simulink library "ammclib_bam_s32k11x"  (Simulink 9.0)
settings: Solver=ode45  StartTime=0.0  StopTime=10.0  RelTol=1e-3
undefined symbols (not defined in the file): f16A1, f16A2, f16B0, f16B1, f16B2, f16C1, f16CC1, f16CC1sc, f16CC1sc_D, f16CC1sc_Q, f16CC1scD, f16CC1scQ, f16CC2, f16CC2sc, f16CC2sc_D, f16CC2sc_Q, f16CC2scD, f16CC2scQ, f16DerivGain, f16EGain, f16FiltCoef, f16HystOff, f16HystOn, f16IGain, f16IntegGain, f16IntegGainFW, f16IntegGainQ, f16Kd, f16Kq, f16Limit, f16LowerLim, f16LowerLimit_D, f16LowerLimit_Q, f16ModIndex, f16OutValOff, f16OutValOn, f16PropGain, f16PropGainFW, f16PropGainQ, f16RampDown, f16RampUp, f16UGain, f16UpperLim, f16UpperLimit, f16UpperLimit_D, f16UpperLimit_Q, f16WIGain, f32A1, f32A2, f32B0, f32B1, f32B2, f32C1, f32CC1, f32CC1sc, f32CC1sc_D, f32CC1sc_Q, f32CC1scD, f32CC1scQ, f32CC2 ... (+71)
(part 6 of 7)

== system ammclib_bam_s32k11x/MLIB/bam_f16/MLIB_AddSat_F16 ==
  note: ---------------------------------------------------------------------------------------------------------------------------------------------------------------------------------------------------
  f16In1 : Inport
  f16In2 : Inport  Port=2
  MLIB_AddSat_SF : S-Function  FunctionName=MLIB_AddSat_SF_F16  SFunctionDeploymentMode=off  EnableBusSupport=off
  copyright : Subsystem
      mask Display:
      | text(10,90,'FILE:');text(10,75,'DESRIPTION:')
      | text(10,60,'COPYRIGHT:')
      | text(10,45,'VERSION:')
      | text(10,30,'DATE:')
  copyright2 : Subsystem
      mask Display:
      | text(10,90,'MLIB_AddSat_BAM_F16.mdl');text(10,75,'Saturated sum of two input values.');text(10,60,'NXP')
      | text(10,45,'0.1');text(10,30,'20-Jan-2012');
  logo : Subsystem
      mask Display: image(imread('logo.jpg'))
  f16Out : Outport
  wires:
  MLIB_AddSat_SF/1 -> f16Out/1
  f16In2/1 -> MLIB_AddSat_SF/2
  f16In1/1 -> MLIB_AddSat_SF/1

== system ammclib_bam_s32k11x/MLIB/bam_f16/MLIB_Add_F16 ==
  note: ---------------------------------------------------------------------------------------------------------------------------------------------------------------------------------------------------
  f16In1 : Inport
  f16In2 : Inport  Port=2
  MLIB_Add_SF : S-Function  FunctionName=MLIB_Add_SF_F16  SFunctionDeploymentMode=off  EnableBusSupport=off
  copyright : Subsystem
      mask Display:
      | text(10,90,'FILE:');text(10,75,'DESRIPTION:')
      | text(10,60,'COPYRIGHT:')
      | text(10,45,'VERSION:')
      | text(10,30,'DATE:')
  copyright2 : Subsystem
      mask Display:
      | text(10,90,'MLIB_Add_BAM_F16.mdl');text(10,75,'Sum of two input values.');text(10,60,'NXP')
      | text(10,45,'0.1');text(10,30,'20-Jan-2012');
  logo : Subsystem
      mask Display: image(imread('logo.jpg'))
  f16Out : Outport
  wires:
  MLIB_Add_SF/1 -> f16Out/1
  f16In2/1 -> MLIB_Add_SF/2
  f16In1/1 -> MLIB_Add_SF/1

== system ammclib_bam_s32k11x/MLIB/bam_f16/MLIB_ConvertPU_F16F32 ==
  note: ---------------------------------------------------------------------------------------------------------------------------------------------------------------------------------------------------
  f32In : Inport
  MLIB_ConvertPU_SF : S-Function  FunctionName=MLIB_ConvertPU_SF_F16F32  SFunctionDeploymentMode=off  EnableBusSupport=off
  copyright : Subsystem
      mask Display: text(10,90,'FILE:');text(10,75,'DESRIPTION:')text(10,60,'COPYRIGHT:')text(10,45,'VERSION:')text(10,30,'DATE:')
  copyright2 : Subsystem
      mask Display: text(10,90,'MLIB_ConvertPU_BAM_F16.mdl');text(10,75,'Converts the input value to different representation in unity model.');text(10,60,'NXP')text(10,45,'0.1');text(10,30,'10-Oct-2011');
  logo : Subsystem
      mask Display: image(imread('logo.jpg'))
  f16Out : Outport
  wires:
  MLIB_ConvertPU_SF/1 -> f16Out/1
  f32In/1 -> MLIB_ConvertPU_SF/1

== system ammclib_bam_s32k11x/MLIB/bam_f16/MLIB_Convert_F16F32 ==
  note: ---------------------------------------------------------------------------------------------------------------------------------------------------------------------------------------------------
  f32In1 : Inport
  f32In2 : Inport  Port=2
  MLIB_Convert_SF : S-Function  FunctionName=MLIB_Convert_SF_F16F32  SFunctionDeploymentMode=off  EnableBusSupport=off
  copyright : Subsystem
      mask Display:
      | text(10,90,'FILE:');text(10,75,'DESRIPTION:')
      | text(10,60,'COPYRIGHT:')
      | text(10,45,'VERSION:')
      | text(10,30,'DATE:')
  copyright2 : Subsystem
      mask Display:
      | text(10,90,'MLIB_Convert_BAM_F16F32.mdl');text(10,75,'Converts the input value with scale to different representation in unity model.');text(10,60,'NXP')
      | text(10,45,'0.1');text(10,30,'13-Oct-2011');
  logo : Subsystem
      mask Display: image(imread('logo.jpg'))
  f16Out : Outport
  wires:
  MLIB_Convert_SF/1 -> f16Out/1
  f32In2/1 -> MLIB_Convert_SF/2
  f32In1/1 -> MLIB_Convert_SF/1

== system ammclib_bam_s32k11x/MLIB/bam_f16/MLIB_DivSat_F16 ==
  note: ---------------------------------------------------------------------------------------------------------------------------------------------------------------------------------------------------
  f16In1 : Inport
  f16In2 : Inport  Port=2
  MLIB_DivSat_SF : S-Function  FunctionName=MLIB_DivSat_SF_F16  SFunctionDeploymentMode=off  EnableBusSupport=off
  copyright : Subsystem
      mask Display:
      | text(10,90,'FILE:');text(10,75,'DESRIPTION:')
      | text(10,60,'COPYRIGHT:')
      | text(10,45,'VERSION:')
      | text(10,30,'DATE:')
  copyright2 : Subsystem
      mask Display:
      | text(10,90,'MLIB_DivSat_BAM_F16.mdl');text(10,75,'Division of two input values saturated if necessary.');text(10,60,'NXP')
      | text(10,45,'0.1');text(10,30,'19-Aug-2011');
  logo : Subsystem
      mask Display: image(imread('logo.jpg'))
  f16Out : Outport
  wires:
  MLIB_DivSat_SF/1 -> f16Out/1
  f16In2/1 -> MLIB_DivSat_SF/2
  f16In1/1 -> MLIB_DivSat_SF/1

== system ammclib_bam_s32k11x/MLIB/bam_f16/MLIB_Div_F16 ==
  note: ---------------------------------------------------------------------------------------------------------------------------------------------------------------------------------------------------
  f16In1 : Inport
  f16In2 : Inport  Port=2
  MLIB_Div_SF : S-Function  FunctionName=MLIB_Div_SF_F16  SFunctionDeploymentMode=off  EnableBusSupport=off
  copyright : Subsystem
      mask Display:
      | text(10,90,'FILE:');text(10,75,'DESRIPTION:')
      | text(10,60,'COPYRIGHT:')
      | text(10,45,'VERSION:')
      | text(10,30,'DATE:')
  copyright2 : Subsystem
      mask Display:
      | text(10,90,'MLIB_Div_BAM_F16.mdl');text(10,75,'Division of two input values.');text(10,60,'Freescale')
      | text(10,45,'0.1');text(10,30,'19-Aug-2011');
  logo : Subsystem
      mask Display: image(imread('logo.jpg'))
  f16Out : Outport
  wires:
  MLIB_Div_SF/1 -> f16Out/1
  f16In2/1 -> MLIB_Div_SF/2
  f16In1/1 -> MLIB_Div_SF/1

== system ammclib_bam_s32k11x/MLIB/bam_f16/MLIB_MacSat_F16 ==
  note: ---------------------------------------------------------------------------------------------------------------------------------------------------------------------------------------------------
  f16In1 : Inport
  f16In2 : Inport  Port=2
  f16In3 : Inport  Port=3
  MLIB_MacSat_SF : S-Function  FunctionName=MLIB_MacSat_SF_F16  SFunctionDeploymentMode=off  EnableBusSupport=off
  copyright : Subsystem
      mask Display:
      | text(10,90,'FILE:');text(10,75,'DESRIPTION:')
      | text(10,60,'COPYRIGHT:')
      | text(10,45,'VERSION:')
      | text(10,30,'DATE:')
  copyright2 : Subsystem
      mask Display:
      | text(10,90,'MLIB_MacSat_BAM_F16.mdl');text(10,75,'Saturated sum of two input values.');text(10,60,'NXP')
      | text(10,45,'0.1');text(10,30,'22-Aug-2011');
  logo : Subsystem
      mask Display: image(imread('logo.jpg'))
  f16Out : Outport
  wires:
  MLIB_MacSat_SF/1 -> f16Out/1
  f16In3/1 -> MLIB_MacSat_SF/3
  f16In2/1 -> MLIB_MacSat_SF/2
  f16In1/1 -> MLIB_MacSat_SF/1

== system ammclib_bam_s32k11x/MLIB/bam_f16/MLIB_Mac_F16 ==
  note: ---------------------------------------------------------------------------------------------------------------------------------------------------------------------------------------------------
  f16In1 : Inport
  f16In2 : Inport  Port=2
  f16In3 : Inport  Port=3
  MLIB_Mac_SF : S-Function  FunctionName=MLIB_Mac_SF_F16  SFunctionDeploymentMode=off  EnableBusSupport=off
  copyright : Subsystem
      mask Display:
      | text(10,90,'FILE:');text(10,75,'DESRIPTION:')
      | text(10,60,'COPYRIGHT:')
      | text(10,45,'VERSION:')
      | text(10,30,'DATE:')
  copyright2 : Subsystem
      mask Display:
      | text(10,90,'MLIB_Mac_BAM_F16.mdl');text(10,75,'Sum of two input values.');text(10,60,'NXP')
      | text(10,45,'0.1');text(10,30,'18-Jul-2011');
  logo : Subsystem
      mask Display: image(imread('logo.jpg'))
  f16Out : Outport
  wires:
  MLIB_Mac_SF/1 -> f16Out/1
  f16In3/1 -> MLIB_Mac_SF/3
  f16In2/1 -> MLIB_Mac_SF/2
  f16In1/1 -> MLIB_Mac_SF/1

== system ammclib_bam_s32k11x/MLIB/bam_f16/MLIB_Mnac_F16 ==
  note: ---------------------------------------------------------------------------------------------------------------------------------------------------------------------------------------------------
  f16In1 : Inport
  f16In2 : Inport  Port=2
  f16In3 : Inport  Port=3
  MLIB_Mnac_SF : S-Function  FunctionName=MLIB_Mnac_SF_F16  SFunctionDeploymentMode=off  EnableBusSupport=off
  copyright : Subsystem
      mask Display:
      | text(10,90,'FILE:');text(10,75,'DESRIPTION:')
      | text(10,60,'COPYRIGHT:')
      | text(10,45,'VERSION:')
      | text(10,30,'DATE:')
  copyright2 : Subsystem
      mask Display:
      | text(10,90,'MLIB_Mnac_BAM_F16.mdl');text(10,75,'Multiply-negative-accumulate.');text(10,60,'Freescale')
      | text(10,45,'1.0');text(10,30,'27-Mar-2015');
  logo : Subsystem
      mask Display: image(imread('logo.jpg'))
  f16Out : Outport
  wires:
  MLIB_Mnac_SF/1 -> f16Out/1
  f16In3/1 -> MLIB_Mnac_SF/3
  f16In2/1 -> MLIB_Mnac_SF/2
  f16In1/1 -> MLIB_Mnac_SF/1

== system ammclib_bam_s32k11x/MLIB/bam_f16/MLIB_Msu_F16 ==
  note: ---------------------------------------------------------------------------------------------------------------------------------------------------------------------------------------------------
  f16In1 : Inport
  f16In2 : Inport  Port=2
  f16In3 : Inport  Port=3
  MLIB_Msu_SF : S-Function  FunctionName=MLIB_Msu_SF_F16  SFunctionDeploymentMode=off  EnableBusSupport=off
  copyright : Subsystem
      mask Display:
      | text(10,90,'FILE:');text(10,75,'DESRIPTION:')
      | text(10,60,'COPYRIGHT:')
      | text(10,45,'VERSION:')
      | text(10,30,'DATE:')
  copyright2 : Subsystem
      mask Display:
      | text(10,90,'MLIB_Msu_BAM_F16.mdl');text(10,75,'Multiply-subtract-from.');text(10,60,'NXP')
      | text(10,45,'1.0');text(10,30,'27-Mar-2015');
  logo : Subsystem
      mask Display: image(imread('logo.jpg'))
  f16Out : Outport
  wires:
  MLIB_Msu_SF/1 -> f16Out/1
  f16In3/1 -> MLIB_Msu_SF/3
  f16In2/1 -> MLIB_Msu_SF/2
  f16In1/1 -> MLIB_Msu_SF/1

== system ammclib_bam_s32k11x/MLIB/bam_f16/MLIB_MulSat_F16 ==
  note: ---------------------------------------------------------------------------------------------------------------------------------------------------------------------------------------------------
  f16In1 : Inport
  f16In2 : Inport  Port=2
  MLIB_MulSat_SF : S-Function  FunctionName=MLIB_MulSat_SF_F16  SFunctionDeploymentMode=off  EnableBusSupport=off
  copyright : Subsystem
      mask Display:
      | text(10,90,'FILE:');text(10,75,'DESRIPTION:')
      | text(10,60,'COPYRIGHT:')
      | text(10,45,'VERSION:')
      | text(10,30,'DATE:')
  copyright2 : Subsystem
      mask Display:
      | text(10,90,'MLIB_MulSat_BAM_F16.mdl');text(10,75,'Saturated sum of two input values.');text(10,60,'NXP')
      | text(10,45,'0.1');text(10,30,'01-Aug-2011');
  logo : Subsystem
      mask Display: image(imread('logo.jpg'))
  f16Out : Outport
  wires:
  MLIB_MulSat_SF/1 -> f16Out/1
  f16In2/1 -> MLIB_MulSat_SF/2
  f16In1/1 -> MLIB_MulSat_SF/1

== system ammclib_bam_s32k11x/MLIB/bam_f16/MLIB_Mul_F16 ==
  note: ---------------------------------------------------------------------------------------------------------------------------------------------------------------------------------------------------
  f16In1 : Inport
  f16In2 : Inport  Port=2
  MLIB_Mul_SF : S-Function  FunctionName=MLIB_Mul_SF_F16  SFunctionDeploymentMode=off  EnableBusSupport=off
  copyright : Subsystem
      mask Display:
      | text(10,90,'FILE:');text(10,75,'DESRIPTION:')
      | text(10,60,'COPYRIGHT:')
      | text(10,45,'VERSION:')
      | text(10,30,'DATE:')
  copyright2 : Subsystem
      mask Display:
      | text(10,90,'MLIB_Mul_BAM_F16.mdl');text(10,75,'Sum of two input values.');text(10,60,'NXP')
      | text(10,45,'0.1');text(10,30,'26-Jul-2011');
  logo : Subsystem
      mask Display: image(imread('logo.jpg'))
  f16Out : Outport
  wires:
  MLIB_Mul_SF/1 -> f16Out/1
  f16In2/1 -> MLIB_Mul_SF/2
  f16In1/1 -> MLIB_Mul_SF/1

== system ammclib_bam_s32k11x/MLIB/bam_f16/MLIB_NegSat_F16 ==
  note: ---------------------------------------------------------------------------------------------------------------------------------------------------------------------------------------------------
  f16In : Inport
  MLIB_NegSat_SF : S-Function  FunctionName=MLIB_NegSat_SF_F16  SFunctionDeploymentMode=off  EnableBusSupport=off
  copyright : Subsystem
      mask Display: text(10,90,'FILE:');text(10,75,'DESRIPTION:')text(10,60,'COPYRIGHT:')text(10,45,'VERSION:')text(10,30,'DATE:')
  copyright2 : Subsystem
      mask Display: text(10,90,'MLIB_NegSat_BAM_F16.mdl');text(10,75,'Sum of two input values.');text(10,60,'NXP')text(10,45,'0.1');text(10,30,'12-Jul-2011');
  logo : Subsystem
      mask Display: image(imread('logo.jpg'))
  f16Out : Outport
  wires:
  MLIB_NegSat_SF/1 -> f16Out/1
  f16In/1 -> MLIB_NegSat_SF/1

== system ammclib_bam_s32k11x/MLIB/bam_f16/MLIB_Neg_F16 ==
  note: ---------------------------------------------------------------------------------------------------------------------------------------------------------------------------------------------------
  f16In : Inport
  MLIB_Neg_SF : S-Function  FunctionName=MLIB_Neg_SF_F16  SFunctionDeploymentMode=off  EnableBusSupport=off
  copyright : Subsystem
      mask Display: text(10,90,'FILE:');text(10,75,'DESRIPTION:')text(10,60,'COPYRIGHT:')text(10,45,'VERSION:')text(10,30,'DATE:')
  copyright2 : Subsystem
      mask Display: text(10,90,'MLIB_Neg_BAM_F16.mdl');text(10,75,'Sum of two input values.');text(10,60,'NXP')text(10,45,'0.1');text(10,30,'20-Jan-2012');
  logo : Subsystem
      mask Display: image(imread('logo.jpg'))
  f16Out : Outport
  wires:
  MLIB_Neg_SF/1 -> f16Out/1
  f16In/1 -> MLIB_Neg_SF/1

== system ammclib_bam_s32k11x/MLIB/bam_f16/MLIB_Norm_F16 ==
  note: ---------------------------------------------------------------------------------------------------------------------------------------------------------------------------------------------------
  f16In : Inport
  MLIB_Norm_SF_F16 : S-Function  FunctionName=MLIB_Norm_SF_F16  SFunctionDeploymentMode=off  EnableBusSupport=off
  copyright : Subsystem
      mask Display: text(10,90,'FILE:');text(10,75,'DESRIPTION:')text(10,60,'COPYRIGHT:')text(10,45,'VERSION:')text(10,30,'DATE:')
  copyright2 : Subsystem
      mask Display: text(10,90,'MLIB_Norm_BAM_F16.mdl');text(10,75,'Normalization of the input value.');text(10,60,'Freescale')text(10,45,'0.1');text(10,30,'15-Sep-2011');
  logo : Subsystem
      mask Display: image(imread('logo.jpg'))
  u16Out : Outport
  wires:
  MLIB_Norm_SF_F16/1 -> u16Out/1
  f16In/1 -> MLIB_Norm_SF_F16/1

== system ammclib_bam_s32k11x/MLIB/bam_f16/MLIB_RndSat_F16F32 ==
  note: ---------------------------------------------------------------------------------------------------------------------------------------------------------------------------------------------------
  f32In : Inport
  MLIB_RndSat_SF : S-Function  FunctionName=MLIB_RndSat_SF_F16F32  SFunctionDeploymentMode=off  EnableBusSupport=off
  copyright : Subsystem
      mask Display: text(10,90,'FILE:');text(10,75,'DESRIPTION:');text(10,60,'COPYRIGHT:');text(10,45,'VERSION:');text(10,30,'DATE:')
  copyright2 : Subsystem
      mask Display: text(10,90,'MLIB_RndSat_BAM_F16F32.mdl');text(10,75,'Rounding of the input value to the nearest saturated value in output format.');text(10,60,'NXP');text(10,45,'1.0');text(10,30,'05-May-2016');
  logo : Subsystem
      mask Display: image(imread('logo.jpg'))
  f16Out : Outport
  wires:
  MLIB_RndSat_SF/1 -> f16Out/1
  f32In/1 -> MLIB_RndSat_SF/1

== system ammclib_bam_s32k11x/MLIB/bam_f16/MLIB_Round_F16 ==
  note: ---------------------------------------------------------------------------------------------------------------------------------------------------------------------------------------------------
  f16In1 : Inport
  u16In2 : Inport  Port=2
  MLIB_Round_SF_F16 : S-Function  FunctionName=MLIB_Round_SF_F16  SFunctionDeploymentMode=off  EnableBusSupport=off
  copyright : Subsystem
      mask Display:
      | text(10,90,'FILE:');text(10,75,'DESRIPTION:')
      | text(10,60,'COPYRIGHT:')
      | text(10,45,'VERSION:')
      | text(10,30,'DATE:')
  copyright2 : Subsystem
      mask Display:
      | text(10,90,'MLIB_Round_BAM_F16.mdl');text(10,75,'Round the first input value.');text(10,60,'Freescale')
      | text(10,45,'0.1');text(10,30,'02-Sep-2011');
  logo : Subsystem
      mask Display: image(imread('logo.jpg'))
  f16Out : Outport
  wires:
  MLIB_Round_SF_F16/1 -> f16Out/1
  u16In2/1 -> MLIB_Round_SF_F16/2
  f16In1/1 -> MLIB_Round_SF_F16/1

== system ammclib_bam_s32k11x/MLIB/bam_f16/MLIB_ShBiSat_F16 ==
  note: ---------------------------------------------------------------------------------------------------------------------------------------------------------------------------------------------------
  f16In1 : Inport
  s16In2 : Inport  Port=2
  MLIB_ShBiSat_SF_F16 : S-Function  FunctionName=MLIB_ShBiSat_SF_F16  SFunctionDeploymentMode=off  EnableBusSupport=off
  copyright : Subsystem
      mask Display:
      | text(10,90,'FILE:');text(10,75,'DESRIPTION:')
      | text(10,60,'COPYRIGHT:')
      | text(10,45,'VERSION:')
      | text(10,30,'DATE:')
  copyright2 : Subsystem
      mask Display:
      | text(10,90,'MLIB_ShBiSat_BAM_F16.mdl');text(10,75,'Shift the first parameter to left or right and saturate if necessary.');text(10,60,'NXP')
      | text(10,45,'0.1');text(10,30,'26-Aug-2011');
  logo : Subsystem
      mask Display: image(imread('logo.jpg'))
  f16Out : Outport
  wires:
  MLIB_ShBiSat_SF_F16/1 -> f16Out/1
  s16In2/1 -> MLIB_ShBiSat_SF_F16/2
  f16In1/1 -> MLIB_ShBiSat_SF_F16/1

== system ammclib_bam_s32k11x/MLIB/bam_f16/MLIB_ShBi_F16 ==
  note: ---------------------------------------------------------------------------------------------------------------------------------------------------------------------------------------------------
  f16In1 : Inport
  s16In2 : Inport  Port=2
  MLIB_ShBi_SF_F16 : S-Function  FunctionName=MLIB_ShBi_SF_F16  SFunctionDeploymentMode=off  EnableBusSupport=off
  copyright : Subsystem
      mask Display:
      | text(10,90,'FILE:');text(10,75,'DESRIPTION:')
      | text(10,60,'COPYRIGHT:')
      | text(10,45,'VERSION:')
      | text(10,30,'DATE:')
  copyright2 : Subsystem
      mask Display:
      | text(10,90,'MLIB_ShBi_BAM_F16.mdl');text(10,75,'Shift the first parameter to left or right.');text(10,60,'NXP')
      | text(10,45,'0.1');text(10,30,'24-Aug-2011');
  logo : Subsystem
      mask Display: image(imread('logo.jpg'))
  f16Out : Outport
  wires:
  MLIB_ShBi_SF_F16/1 -> f16Out/1
  s16In2/1 -> MLIB_ShBi_SF_F16/2
  f16In1/1 -> MLIB_ShBi_SF_F16/1

== system ammclib_bam_s32k11x/MLIB/bam_f16/MLIB_ShLSat_F16 ==
  note: ---------------------------------------------------------------------------------------------------------------------------------------------------------------------------------------------------
  f16In1 : Inport
  u16In2 : Inport  Port=2
  MLIB_ShLSat_SF : S-Function  FunctionName=MLIB_ShLSat_SF_F16  SFunctionDeploymentMode=off  EnableBusSupport=off
  copyright : Subsystem
      mask Display:
      | text(10,90,'FILE:');text(10,75,'DESRIPTION:')
      | text(10,60,'COPYRIGHT:')
      | text(10,45,'VERSION:')
      | text(10,30,'DATE:')
  copyright2 : Subsystem
      mask Display:
      | text(10,90,'MLIB_ShLSat_BAM_F16.mdl');text(10,75,'Shift the first parameter to left and saturate if necessary.');text(10,60,'NXP')
      | text(10,45,'0.1');text(10,30,'19-Jul-2011');
  logo : Subsystem
      mask Display: image(imread('logo.jpg'))
  f16Out : Outport
  wires:
  MLIB_ShLSat_SF/1 -> f16Out/1
  u16In2/1 -> MLIB_ShLSat_SF/2
  f16In1/1 -> MLIB_ShLSat_SF/1

== system ammclib_bam_s32k11x/MLIB/bam_f16/MLIB_ShL_F16 ==
  note: ---------------------------------------------------------------------------------------------------------------------------------------------------------------------------------------------------
  f16In1 : Inport
  u16In2 : Inport  Port=2
  MLIB_ShL_SF_F16 : S-Function  FunctionName=MLIB_ShL_SF_F16  SFunctionDeploymentMode=off  EnableBusSupport=off
  copyright : Subsystem
      mask Display:
      | text(10,90,'FILE:');text(10,75,'DESRIPTION:')
      | text(10,60,'COPYRIGHT:')
      | text(10,45,'VERSION:')
      | text(10,30,'DATE:')
      | text(10,15,'AUTHOR:')
  copyright2 : Subsystem
      mask Display:
      | text(10,90,'MLIB_ShL_BAM_F16.mdl');text(10,75,'Shift the first parameter to left.');text(10,60,'Freescale')
      | text(10,45,'0.1');text(10,30,'04-Jul-2011');text(10,15,'');
  logo : Subsystem
      mask Display: image(imread('logo.jpg'))
  f16Out : Outport
  wires:
  u16In2/1 -> MLIB_ShL_SF_F16/2
  MLIB_ShL_SF_F16/1 -> f16Out/1
  f16In1/1 -> MLIB_ShL_SF_F16/1

== system ammclib_bam_s32k11x/MLIB/bam_f16/MLIB_ShR_F16 ==
  note: ---------------------------------------------------------------------------------------------------------------------------------------------------------------------------------------------------
  f16In1 : Inport
  u16In2 : Inport  Port=2
  MLIB_ShR_SF : S-Function  FunctionName=MLIB_ShR_SF_F16  SFunctionDeploymentMode=off  EnableBusSupport=off
  copyright : Subsystem
      mask Display:
      | text(10,90,'FILE:');text(10,75,'DESRIPTION:')
      | text(10,60,'COPYRIGHT:')
      | text(10,45,'VERSION:')
      | text(10,30,'DATE:')
  copyright2 : Subsystem
      mask Display:
      | text(10,90,'MLIB_ShR_BAM_F16.mdl');text(10,75,'Shift the first parameter to right.');text(10,60,'Freescale')
      | text(10,45,'0.1');text(10,30,'20-Jul-2011');
  logo : Subsystem
      mask Display: image(imread('logo.jpg'))
  f16Out : Outport
  wires:
  MLIB_ShR_SF/1 -> f16Out/1
  u16In2/1 -> MLIB_ShR_SF/2
  f16In1/1 -> MLIB_ShR_SF/1

== system ammclib_bam_s32k11x/MLIB/bam_f16/MLIB_SubSat_F16 ==
  note: ---------------------------------------------------------------------------------------------------------------------------------------------------------------------------------------------------
  f16In1 : Inport
  f16In2 : Inport  Port=2
  MLIB_SubSat_SF : S-Function  FunctionName=MLIB_SubSat_SF_F16  SFunctionDeploymentMode=off  EnableBusSupport=off
  copyright : Subsystem
      mask Display:
      | text(10,90,'FILE:');text(10,75,'DESRIPTION:')
      | text(10,60,'COPYRIGHT:')
      | text(10,45,'VERSION:')
      | text(10,30,'DATE:')
  copyright2 : Subsystem
      mask Display:
      | text(10,90,'MLIB_SubSat_BAM_F16.mdl');text(10,75,'Saturated sum of two input values.');text(10,60,'NXP')
      | text(10,45,'0.1');text(10,30,'20-Jan-2012');
  logo : Subsystem
      mask Display: image(imread('logo.jpg'))
  f16Out : Outport
  wires:
  MLIB_SubSat_SF/1 -> f16Out/1
  f16In2/1 -> MLIB_SubSat_SF/2
  f16In1/1 -> MLIB_SubSat_SF/1

== system ammclib_bam_s32k11x/MLIB/bam_f16/MLIB_Sub_F16 ==
  note: ---------------------------------------------------------------------------------------------------------------------------------------------------------------------------------------------------
  f16In1 : Inport
  f16In2 : Inport  Port=2
  MLIB_Sub_SF : S-Function  FunctionName=MLIB_Sub_SF_F16  SFunctionDeploymentMode=off  EnableBusSupport=off
  copyright : Subsystem
      mask Display:
      | text(10,90,'FILE:');text(10,75,'DESRIPTION:')
      | text(10,60,'COPYRIGHT:')
      | text(10,45,'VERSION:')
      | text(10,30,'DATE:')
  copyright2 : Subsystem
      mask Display:
      | text(10,90,'MLIB_Sub_BAM_F16.mdl');text(10,75,'Sum of two input values.');text(10,60,'NXP')
      | text(10,45,'0.1');text(10,30,'18-Jul-2011');
  logo : Subsystem
      mask Display: image(imread('logo.jpg'))
  f16Out : Outport
  wires:
  MLIB_Sub_SF/1 -> f16Out/1
  f16In2/1 -> MLIB_Sub_SF/2
  f16In1/1 -> MLIB_Sub_SF/1

== system ammclib_bam_s32k11x/MLIB/bam_f16/MLIB_VMac_F16 ==
  note: ---------------------------------------------------------------------------------------------------------------------------------------------------------------------------------------------------
  f16In1 : Inport
  f16In2 : Inport  Port=2
  f16In3 : Inport  Port=3
  f16In4 : Inport  Port=4
  MLIB_VMac_SF : S-Function  FunctionName=MLIB_VMac_SF_F16  SFunctionDeploymentMode=off  EnableBusSupport=off
  copyright : Subsystem
      mask Display:
      | text(10,90,'FILE:');text(10,75,'DESRIPTION:')
      | text(10,60,'COPYRIGHT:')
      | text(10,45,'VERSION:')
      | text(10,30,'DATE:')
  copyright2 : Subsystem
      mask Display:
      | text(10,90,'MLIB_VMac_BAM_F16.mdl');text(10,75,'Vector multiply accumulate.');text(10,60,'Freescale')
      | text(10,45,'0.1');text(10,30,'25-Aug-2011');
  logo : Subsystem
      mask Display: image(imread('logo.jpg'))
  f16Out : Outport
  wires:
  MLIB_VMac_SF/1 -> f16Out/1
  f16In4/1 -> MLIB_VMac_SF/4
  f16In3/1 -> MLIB_VMac_SF/3
  f16In2/1 -> MLIB_VMac_SF/2
  f16In1/1 -> MLIB_VMac_SF/1

== system ammclib_bam_s32k11x/MLIB/bam_f32/MLIB_AbsSat_F32 ==
  note: ---------------------------------------------------------------------------------------------------------------------------------------------------------------------------------------------------
  f32In : Inport
  MLIB_AbsSat_SF : S-Function  FunctionName=MLIB_AbsSat_SF_F32  SFunctionDeploymentMode=off  EnableBusSupport=off
  copyright : Subsystem
      mask Display: text(10,90,'FILE:');text(10,75,'DESRIPTION:')text(10,60,'COPYRIGHT:')text(10,45,'VERSION:')text(10,30,'DATE:')
  copyright2 : Subsystem
      mask Display: text(10,90,'MLIB_AbsSat_BAM_F32.mdl');text(10,75,'Absolute value of input parameter saturated if necessary.');text(10,60,'NXP')text(10,45,'0.1');text(10,30,'19-Aug-2011');
  logo : Subsystem
      mask Display: image(imread('logo.jpg'))
  f32Out : Outport
  wires:
  MLIB_AbsSat_SF/1 -> f32Out/1
  f32In/1 -> MLIB_AbsSat_SF/1

== system ammclib_bam_s32k11x/MLIB/bam_f32/MLIB_Abs_F32 ==
  note: ---------------------------------------------------------------------------------------------------------------------------------------------------------------------------------------------------
  f32In : Inport
  MLIB_Abs_SF : S-Function  FunctionName=MLIB_Abs_SF_F32  SFunctionDeploymentMode=off  EnableBusSupport=off
  copyright : Subsystem
      mask Display: text(10,90,'FILE:');text(10,75,'DESRIPTION:')text(10,60,'COPYRIGHT:')text(10,45,'VERSION:')text(10,30,'DATE:')
  copyright2 : Subsystem
      mask Display: text(10,90,'MLIB_Abs_BAM_F32.mdl');text(10,75,'Absolute value of input parameter.');text(10,60,'Freescale')text(10,45,'0.1');text(10,30,'20-Jan-2012');
  logo : Subsystem
      mask Display: image(imread('logo.jpg'))
  f32Out : Outport
  wires:
  MLIB_Abs_SF/1 -> f32Out/1
  f32In/1 -> MLIB_Abs_SF/1

== system ammclib_bam_s32k11x/MLIB/bam_f32/MLIB_AddSat_F32 ==
  note: ---------------------------------------------------------------------------------------------------------------------------------------------------------------------------------------------------
  f32In1 : Inport
  f32In2 : Inport  Port=2
  MLIB_AddSat_SF : S-Function  FunctionName=MLIB_AddSat_SF_F32  SFunctionDeploymentMode=off  EnableBusSupport=off
  copyright : Subsystem
      mask Display:
      | text(10,90,'FILE:');text(10,75,'DESRIPTION:')
      | text(10,60,'COPYRIGHT:')
      | text(10,45,'VERSION:')
      | text(10,30,'DATE:')
  copyright2 : Subsystem
      mask Display:
      | text(10,90,'MLIB_AddSat_BAM_F32.mdl');text(10,75,'Saturated sum of two input values.');text(10,60,'NXP')
      | text(10,45,'0.1');text(10,30,'20-Jan-2012');
  logo : Subsystem
      mask Display: image(imread('logo.jpg'))
  f32Out : Outport
  wires:
  MLIB_AddSat_SF/1 -> f32Out/1
  f32In2/1 -> MLIB_AddSat_SF/2
  f32In1/1 -> MLIB_AddSat_SF/1

== system ammclib_bam_s32k11x/MLIB/bam_f32/MLIB_Add_F32 ==
  note: ---------------------------------------------------------------------------------------------------------------------------------------------------------------------------------------------------
  f32In1 : Inport
  f32In2 : Inport  Port=2
  MLIB_Add_SF : S-Function  FunctionName=MLIB_Add_SF_F32  SFunctionDeploymentMode=off  EnableBusSupport=off
  copyright : Subsystem
      mask Display:
      | text(10,90,'FILE:');text(10,75,'DESRIPTION:')
      | text(10,60,'COPYRIGHT:')
      | text(10,45,'VERSION:')
      | text(10,30,'DATE:')
  copyright2 : Subsystem
      mask Display:
      | text(10,90,'MLIB_Add_BAM_F32.mdl');text(10,75,'Sum of two input values.');text(10,60,'NXP')
      | text(10,45,'0.1');text(10,30,'20-Jan-2012');
  logo : Subsystem
      mask Display: image(imread('logo.jpg'))
  f32Out : Outport
  wires:
  MLIB_Add_SF/1 -> f32Out/1
  f32In2/1 -> MLIB_Add_SF/2
  f32In1/1 -> MLIB_Add_SF/1

== system ammclib_bam_s32k11x/MLIB/bam_f32/MLIB_ConvertPU_F32F16 ==
  note: ---------------------------------------------------------------------------------------------------------------------------------------------------------------------------------------------------
  f16In : Inport
  MLIB_ConvertPU_SF : S-Function  FunctionName=MLIB_ConvertPU_SF_F32F16  SFunctionDeploymentMode=off  EnableBusSupport=off
  copyright : Subsystem
      mask Display: text(10,90,'FILE:');text(10,75,'DESRIPTION:')text(10,60,'COPYRIGHT:')text(10,45,'VERSION:')text(10,30,'DATE:')
  copyright2 : Subsystem
      mask Display: text(10,90,'MLIB_ConvertPU_BAM_F32.mdl');text(10,75,'Converts the input value to different representation in unity model.');text(10,60,'NXP')text(10,45,'0.1');text(10,30,'10-Oct-2011');
  logo : Subsystem
      mask Display: image(imread('logo.jpg'))
  f32Out : Outport
  wires:
  MLIB_ConvertPU_SF/1 -> f32Out/1
  f16In/1 -> MLIB_ConvertPU_SF/1

== system ammclib_bam_s32k11x/MLIB/bam_f32/MLIB_Convert_F32F16 ==
  note: ---------------------------------------------------------------------------------------------------------------------------------------------------------------------------------------------------
  f16In1 : Inport
  f16In2 : Inport  Port=2
  MLIB_Convert_SF : S-Function  FunctionName=MLIB_Convert_SF_F32F16  SFunctionDeploymentMode=off  EnableBusSupport=off
  copyright : Subsystem
      mask Display:
      | text(10,90,'FILE:');text(10,75,'DESRIPTION:')
      | text(10,60,'COPYRIGHT:')
      | text(10,45,'VERSION:')
      | text(10,30,'DATE:')
  copyright2 : Subsystem
      mask Display:
      | text(10,90,'MLIB_Convert_BAM_F32F16.mdl');text(10,75,'Converts the input value with scale to different representation in unity model.');text(10,60,'NXP')
      | text(10,45,'0.1');text(10,30,'13-Oct-2011');
  logo : Subsystem
      mask Display: image(imread('logo.jpg'))
  f32Out : Outport
  wires:
  MLIB_Convert_SF/1 -> f32Out/1
  f16In2/1 -> MLIB_Convert_SF/2
  f16In1/1 -> MLIB_Convert_SF/1

== system ammclib_bam_s32k11x/MLIB/bam_f32/MLIB_DivSat_F32 ==
  note: ---------------------------------------------------------------------------------------------------------------------------------------------------------------------------------------------------
  f32In1 : Inport
  f32In2 : Inport  Port=2
  MLIB_DivSat_SF : S-Function  FunctionName=MLIB_DivSat_SF_F32  SFunctionDeploymentMode=off  EnableBusSupport=off
  copyright : Subsystem
      mask Display:
      | text(10,90,'FILE:');text(10,75,'DESRIPTION:')
      | text(10,60,'COPYRIGHT:')
      | text(10,45,'VERSION:')
      | text(10,30,'DATE:')
  copyright2 : Subsystem
      mask Display:
      | text(10,90,'MLIB_DivSat_BAM_F32.mdl');text(10,75,'Division of two input values saturated if necessary.');text(10,60,'NXP')
      | text(10,45,'0.1');text(10,30,'19-Aug-2011');
  logo : Subsystem
      mask Display: image(imread('logo.jpg'))
  f32Out : Outport
  wires:
  MLIB_DivSat_SF/1 -> f32Out/1
  f32In2/1 -> MLIB_DivSat_SF/2
  f32In1/1 -> MLIB_DivSat_SF/1

== system ammclib_bam_s32k11x/MLIB/bam_f32/MLIB_Div_F32 ==
  note: ---------------------------------------------------------------------------------------------------------------------------------------------------------------------------------------------------
  f32In1 : Inport
  f32In2 : Inport  Port=2
  MLIB_Div_SF : S-Function  FunctionName=MLIB_Div_SF_F32  SFunctionDeploymentMode=off  EnableBusSupport=off
  copyright : Subsystem
      mask Display:
      | text(10,90,'FILE:');text(10,75,'DESRIPTION:')
      | text(10,60,'COPYRIGHT:')
      | text(10,45,'VERSION:')
      | text(10,30,'DATE:')
  copyright2 : Subsystem
      mask Display:
      | text(10,90,'MLIB_Div_BAM_F32.mdl');text(10,75,'Division of two input values.');text(10,60,'Freescale')
      | text(10,45,'0.1');text(10,30,'19-Aug-2011');
  logo : Subsystem
      mask Display: image(imread('logo.jpg'))
  f32Out : Outport
  wires:
  MLIB_Div_SF/1 -> f32Out/1
  f32In2/1 -> MLIB_Div_SF/2
  f32In1/1 -> MLIB_Div_SF/1

== system ammclib_bam_s32k11x/MLIB/bam_f32/MLIB_MacSat_F32 ==
  note: ---------------------------------------------------------------------------------------------------------------------------------------------------------------------------------------------------
  f32In1 : Inport
  f32In2 : Inport  Port=2
  f32In3 : Inport  Port=3
  MLIB_MacSat_SF : S-Function  FunctionName=MLIB_MacSat_SF_F32  SFunctionDeploymentMode=off  EnableBusSupport=off
  copyright : Subsystem
      mask Display:
      | text(10,90,'FILE:');text(10,75,'DESRIPTION:')
      | text(10,60,'COPYRIGHT:')
      | text(10,45,'VERSION:')
      | text(10,30,'DATE:')
  copyright2 : Subsystem
      mask Display:
      | text(10,90,'MLIB_MacSat_BAM_F32.mdl');text(10,75,'Multiplication of second and third input value and adding of first input value, staturated if necessary.');text(10,60,'NXP')
      | text(10,45,'0.1');text(10,30,'22-Aug-2011');
  logo : Subsystem
      mask Display: image(imread('logo.jpg'))
  f32Out : Outport
  wires:
  MLIB_MacSat_SF/1 -> f32Out/1
  f32In3/1 -> MLIB_MacSat_SF/3
  f32In2/1 -> MLIB_MacSat_SF/2
  f32In1/1 -> MLIB_MacSat_SF/1

== system ammclib_bam_s32k11x/MLIB/bam_f32/MLIB_Mac_F32 ==
  note: ---------------------------------------------------------------------------------------------------------------------------------------------------------------------------------------------------
  f32In1 : Inport
  f32In2 : Inport  Port=2
  f32In3 : Inport  Port=3
  MLIB_Mac_SF : S-Function  FunctionName=MLIB_Mac_SF_F32  SFunctionDeploymentMode=off  EnableBusSupport=off
  copyright : Subsystem
      mask Display:
      | text(10,90,'FILE:');text(10,75,'DESRIPTION:')
      | text(10,60,'COPYRIGHT:')
      | text(10,45,'VERSION:')
      | text(10,30,'DATE:')
  copyright2 : Subsystem
      mask Display:
      | text(10,90,'MLIB_Mac_BAM_F32.mdl');text(10,75,'Sum of two input values.');text(10,60,'NXP')
      | text(10,45,'0.1');text(10,30,'18-Jul-2011');
  logo : Subsystem
      mask Display: image(imread('logo.jpg'))
  f32Out : Outport
  wires:
  MLIB_Mac_SF/1 -> f32Out/1
  f32In3/1 -> MLIB_Mac_SF/3
  f32In2/1 -> MLIB_Mac_SF/2
  f32In1/1 -> MLIB_Mac_SF/1

== system ammclib_bam_s32k11x/MLIB/bam_f32/MLIB_Mnac_F32 ==
  note: ---------------------------------------------------------------------------------------------------------------------------------------------------------------------------------------------------
  f32In1 : Inport
  f32In2 : Inport  Port=2
  f32In3 : Inport  Port=3
  MLIB_Mnac_SF : S-Function  FunctionName=MLIB_Mnac_SF_F32  SFunctionDeploymentMode=off  EnableBusSupport=off
  copyright : Subsystem
      mask Display:
      | text(10,90,'FILE:');text(10,75,'DESRIPTION:')
      | text(10,60,'COPYRIGHT:')
      | text(10,45,'VERSION:')
      | text(10,30,'DATE:')
  copyright2 : Subsystem
      mask Display:
      | text(10,90,'MLIB_Mnac_BAM_F32.mdl');text(10,75,'Multiply-negative-accumulate.');text(10,60,'Freescale')
      | text(10,45,'1.0');text(10,30,'27-Mar-2015');
  logo : Subsystem
      mask Display: image(imread('logo.jpg'))
  f32Out : Outport
  wires:
  MLIB_Mnac_SF/1 -> f32Out/1
  f32In3/1 -> MLIB_Mnac_SF/3
  f32In2/1 -> MLIB_Mnac_SF/2
  f32In1/1 -> MLIB_Mnac_SF/1

== system ammclib_bam_s32k11x/MLIB/bam_f32/MLIB_Msu_F32 ==
  note: ---------------------------------------------------------------------------------------------------------------------------------------------------------------------------------------------------
  f32In1 : Inport
  f32In2 : Inport  Port=2
  f32In3 : Inport  Port=3
  MLIB_Msu_SF : S-Function  FunctionName=MLIB_Msu_SF_F32  SFunctionDeploymentMode=off  EnableBusSupport=off
  copyright : Subsystem
      mask Display:
      | text(10,90,'FILE:');text(10,75,'DESRIPTION:')
      | text(10,60,'COPYRIGHT:')
      | text(10,45,'VERSION:')
      | text(10,30,'DATE:')
  copyright2 : Subsystem
      mask Display:
      | text(10,90,'MLIB_Msu_BAM_F32.mdl');text(10,75,'Multiply-subtract-from.');text(10,60,'NXP')
      | text(10,45,'1.0');text(10,30,'27-Mar-2015');
  logo : Subsystem
      mask Display: image(imread('logo.jpg'))
  f32Out : Outport
  wires:
  MLIB_Msu_SF/1 -> f32Out/1
  f32In3/1 -> MLIB_Msu_SF/3
  f32In2/1 -> MLIB_Msu_SF/2
  f32In1/1 -> MLIB_Msu_SF/1

== system ammclib_bam_s32k11x/MLIB/bam_f32/MLIB_MulSat_F32 ==
  note: ---------------------------------------------------------------------------------------------------------------------------------------------------------------------------------------------------
  f32In1 : Inport
  f32In2 : Inport  Port=2
  MLIB_MulSat_SF : S-Function  FunctionName=MLIB_MulSat_SF_F32  SFunctionDeploymentMode=off  EnableBusSupport=off
  copyright : Subsystem
      mask Display:
      | text(10,90,'FILE:');text(10,75,'DESRIPTION:')
      | text(10,60,'COPYRIGHT:')
      | text(10,45,'VERSION:')
      | text(10,30,'DATE:')
  copyright2 : Subsystem
      mask Display:
      | text(10,90,'MLIB_MulSat_BAM_F32.mdl');text(10,75,'Saturated sum of two input values.');text(10,60,'NXP')
      | text(10,45,'0.1');text(10,30,'01-Aug-2011');
  logo : Subsystem
      mask Display: image(imread('logo.jpg'))
  f32Out : Outport
  wires:
  MLIB_MulSat_SF/1 -> f32Out/1
  f32In2/1 -> MLIB_MulSat_SF/2
  f32In1/1 -> MLIB_MulSat_SF/1

== system ammclib_bam_s32k11x/MLIB/bam_f32/MLIB_Mul_F32 ==
  note: ---------------------------------------------------------------------------------------------------------------------------------------------------------------------------------------------------
  f32In1 : Inport
  f32In2 : Inport  Port=2
  MLIB_Mul_SF : S-Function  FunctionName=MLIB_Mul_SF_F32  SFunctionDeploymentMode=off  EnableBusSupport=off
  copyright : Subsystem
      mask Display:
      | text(10,90,'FILE:');text(10,75,'DESRIPTION:')
      | text(10,60,'COPYRIGHT:')
      | text(10,45,'VERSION:')
      | text(10,30,'DATE:')
  copyright2 : Subsystem
      mask Display:
      | text(10,90,'MLIB_Mul_BAM_F32.mdl');text(10,75,'Sum of two input values.');text(10,60,'NXP')
      | text(10,45,'0.1');text(10,30,'26-Jul-2011');
  logo : Subsystem
      mask Display: image(imread('logo.jpg'))
  f32Out : Outport
  wires:
  MLIB_Mul_SF/1 -> f32Out/1
  f32In2/1 -> MLIB_Mul_SF/2
  f32In1/1 -> MLIB_Mul_SF/1

== system ammclib_bam_s32k11x/MLIB/bam_f32/MLIB_NegSat_F32 ==
  note: ---------------------------------------------------------------------------------------------------------------------------------------------------------------------------------------------------
  f32In : Inport
  MLIB_NegSat_SF : S-Function  FunctionName=MLIB_NegSat_SF_F32  SFunctionDeploymentMode=off  EnableBusSupport=off
  copyright : Subsystem
      mask Display: text(10,90,'FILE:');text(10,75,'DESRIPTION:')text(10,60,'COPYRIGHT:')text(10,45,'VERSION:')text(10,30,'DATE:')
  copyright2 : Subsystem
      mask Display: text(10,90,'MLIB_NegSat_BAM_F32.mdl');text(10,75,'Sum of two input values.');text(10,60,'NXP')text(10,45,'0.1');text(10,30,'12-Jul-2011');
  logo : Subsystem
      mask Display: image(imread('logo.jpg'))
  f32Out : Outport
  wires:
  MLIB_NegSat_SF/1 -> f32Out/1
  f32In/1 -> MLIB_NegSat_SF/1

== system ammclib_bam_s32k11x/MLIB/bam_f32/MLIB_Neg_F32 ==
  note: ---------------------------------------------------------------------------------------------------------------------------------------------------------------------------------------------------
  f32In : Inport
  MLIB_Neg_SF : S-Function  FunctionName=MLIB_Neg_SF_F32  SFunctionDeploymentMode=off  EnableBusSupport=off
  copyright : Subsystem
      mask Display: text(10,90,'FILE:');text(10,75,'DESRIPTION:')text(10,60,'COPYRIGHT:')text(10,45,'VERSION:')text(10,30,'DATE:')
  copyright2 : Subsystem
      mask Display: text(10,90,'MLIB_Neg_BAM_F32.mdl');text(10,75,'Sum of two input values.');text(10,60,'NXP')text(10,45,'0.1');text(10,30,'20-Jan-2012');
  logo : Subsystem
      mask Display: image(imread('logo.jpg'))
  f32Out : Outport
  wires:
  MLIB_Neg_SF/1 -> f32Out/1
  f32In/1 -> MLIB_Neg_SF/1

== system ammclib_bam_s32k11x/MLIB/bam_f32/MLIB_Norm_F32 ==
  note: ---------------------------------------------------------------------------------------------------------------------------------------------------------------------------------------------------
  f32In : Inport
  MLIB_Norm_SF_F32 : S-Function  FunctionName=MLIB_Norm_SF_F32  SFunctionDeploymentMode=off  EnableBusSupport=off
  copyright : Subsystem
      mask Display:
      | text(10,90,'FILE:');text(10,75,'DESRIPTION:')
      | text(10,60,'COPYRIGHT:')
      | text(10,45,'VERSION:')
      | text(10,30,'DATE:')
  copyright2 : Subsystem
      mask Display:
      | text(10,90,'MLIB_Norm_BAM_F32.mdl');text(10,75,'Normalization of the input value.');text(10,60,'Freescale')
      | text(10,45,'0.1');text(10,30,'15-Sep-2011');
  logo : Subsystem
      mask Display: image(imread('logo.jpg'))
  u16Out : Outport
  wires:
  MLIB_Norm_SF_F32/1 -> u16Out/1
  f32In/1 -> MLIB_Norm_SF_F32/1

== system ammclib_bam_s32k11x/MLIB/bam_f32/MLIB_Round_F32 ==
  note: ---------------------------------------------------------------------------------------------------------------------------------------------------------------------------------------------------
  f32In1 : Inport
  u16In2 : Inport  Port=2
  MLIB_Round_SF_F32 : S-Function  FunctionName=MLIB_Round_SF_F32  SFunctionDeploymentMode=off  EnableBusSupport=off
  copyright : Subsystem
      mask Display:
      | text(10,90,'FILE:');text(10,75,'DESRIPTION:')
      | text(10,60,'COPYRIGHT:')
      | text(10,45,'VERSION:')
      | text(10,30,'DATE:')
  copyright2 : Subsystem
      mask Display:
      | text(10,90,'MLIB_Round_BAM_F32.mdl');text(10,75,'Round the first input value.');text(10,60,'Freescale')
      | text(10,45,'0.1');text(10,30,'02-Sep-2011');
  logo : Subsystem
      mask Display: image(imread('logo.jpg'))
  f32Out : Outport
  wires:
  MLIB_Round_SF_F32/1 -> f32Out/1
  u16In2/1 -> MLIB_Round_SF_F32/2
  f32In1/1 -> MLIB_Round_SF_F32/1

== system ammclib_bam_s32k11x/MLIB/bam_f32/MLIB_ShBiSat_F32 ==
  note: ---------------------------------------------------------------------------------------------------------------------------------------------------------------------------------------------------
  f32In1 : Inport
  s16In2 : Inport  Port=2
  MLIB_ShBiSat_SF_F32 : S-Function  FunctionName=MLIB_ShBiSat_SF_F32  SFunctionDeploymentMode=off  EnableBusSupport=off
  copyright : Subsystem
      mask Display:
      | text(10,90,'FILE:');text(10,75,'DESRIPTION:')
      | text(10,60,'COPYRIGHT:')
      | text(10,45,'VERSION:')
      | text(10,30,'DATE:')
  copyright2 : Subsystem
      mask Display:
      | text(10,90,'MLIB_ShBiSat_BAM_F32.mdl');text(10,75,'Shift the first parameter to left or right and saturate if necessary.');text(10,60,'NXP')
      | text(10,45,'0.1');text(10,30,'26-Aug-2011');
  logo : Subsystem
      mask Display: image(imread('logo.jpg'))
  f32Out : Outport
  wires:
  MLIB_ShBiSat_SF_F32/1 -> f32Out/1
  s16In2/1 -> MLIB_ShBiSat_SF_F32/2
  f32In1/1 -> MLIB_ShBiSat_SF_F32/1

== system ammclib_bam_s32k11x/MLIB/bam_f32/MLIB_ShBi_F32 ==
  note: ---------------------------------------------------------------------------------------------------------------------------------------------------------------------------------------------------
  f32In1 : Inport
  s16In2 : Inport  Port=2
  MLIB_ShBi_SF_F32 : S-Function  FunctionName=MLIB_ShBi_SF_F32  SFunctionDeploymentMode=off  EnableBusSupport=off
  copyright : Subsystem
      mask Display:
      | text(10,90,'FILE:');text(10,75,'DESRIPTION:')
      | text(10,60,'COPYRIGHT:')
      | text(10,45,'VERSION:')
      | text(10,30,'DATE:')
  copyright2 : Subsystem
      mask Display:
      | text(10,90,'MLIB_ShBi_BAM_F32.mdl');text(10,75,'Shift the first parameter to left or right.');text(10,60,'NXP')
      | text(10,45,'0.1');text(10,30,'24-Aug-2011');
  logo : Subsystem
      mask Display: image(imread('logo.jpg'))
  f32Out : Outport
  wires:
  MLIB_ShBi_SF_F32/1 -> f32Out/1
  s16In2/1 -> MLIB_ShBi_SF_F32/2
  f32In1/1 -> MLIB_ShBi_SF_F32/1

== system ammclib_bam_s32k11x/MLIB/bam_f32/MLIB_ShLSat_F32 ==
  note: ---------------------------------------------------------------------------------------------------------------------------------------------------------------------------------------------------
  f32In1 : Inport
  u16In2 : Inport  Port=2
  MLIB_ShLSat_SF : S-Function  FunctionName=MLIB_ShLSat_SF_F32  SFunctionDeploymentMode=off  EnableBusSupport=off
  copyright : Subsystem
      mask Display:
      | text(10,90,'FILE:');text(10,75,'DESRIPTION:')
      | text(10,60,'COPYRIGHT:')
      | text(10,45,'VERSION:')
      | text(10,30,'DATE:')
  copyright2 : Subsystem
      mask Display:
      | text(10,90,'MLIB_ShLSat_BAM_F32.mdl');text(10,75,'Shift the first parameter to left and saturate if necessary.');text(10,60,'NXP')
      | text(10,45,'0.1');text(10,30,'19-Jul-2011');
  logo : Subsystem
      mask Display: image(imread('logo.jpg'))
  f32Out : Outport
  wires:
  MLIB_ShLSat_SF/1 -> f32Out/1
  u16In2/1 -> MLIB_ShLSat_SF/2
  f32In1/1 -> MLIB_ShLSat_SF/1

== system ammclib_bam_s32k11x/MLIB/bam_f32/MLIB_ShL_F32 ==
  note: ---------------------------------------------------------------------------------------------------------------------------------------------------------------------------------------------------
  f32In1 : Inport
  u16In2 : Inport  Port=2
  MLIB_ShL_SF_F32 : S-Function  FunctionName=MLIB_ShL_SF_F32  SFunctionDeploymentMode=off  EnableBusSupport=off
  copyright : Subsystem
      mask Display:
      | text(10,90,'FILE:');text(10,75,'DESRIPTION:')
      | text(10,60,'COPYRIGHT:')
      | text(10,45,'VERSION:')
      | text(10,30,'DATE:')
      | text(10,15,'AUTHOR:')
  copyright2 : Subsystem
      mask Display:
      | text(10,90,'MLIB_ShL_BAM_F32.mdl');text(10,75,'Shift the first parameter to left.');text(10,60,'Freescale')
      | text(10,45,'0.1');text(10,30,'04-Jul-2011');text(10,15,'');
  logo : Subsystem
      mask Display: image(imread('logo.jpg'))
  f32Out : Outport
  wires:
  f32In1/1 -> MLIB_ShL_SF_F32/1
  u16In2/1 -> MLIB_ShL_SF_F32/2
  MLIB_ShL_SF_F32/1 -> f32Out/1

== system ammclib_bam_s32k11x/MLIB/bam_f32/MLIB_ShR_F32 ==
  note: ---------------------------------------------------------------------------------------------------------------------------------------------------------------------------------------------------
  f32In1 : Inport
  u16In2 : Inport  Port=2
  MLIB_ShR_SF : S-Function  FunctionName=MLIB_ShR_SF_F32  SFunctionDeploymentMode=off  EnableBusSupport=off
  copyright : Subsystem
      mask Display:
      | text(10,90,'FILE:');text(10,75,'DESRIPTION:')
      | text(10,60,'COPYRIGHT:')
      | text(10,45,'VERSION:')
      | text(10,30,'DATE:')
  copyright2 : Subsystem
      mask Display:
      | text(10,90,'MLIB_ShR_BAM_F32.mdl');text(10,75,'Shift the first parameter to right.');text(10,60,'Freescale')
      | text(10,45,'0.1');text(10,30,'20-Jul-2011');
  logo : Subsystem
      mask Display: image(imread('logo.jpg'))
  f32Out : Outport
  wires:
  MLIB_ShR_SF/1 -> f32Out/1
  u16In2/1 -> MLIB_ShR_SF/2
  f32In1/1 -> MLIB_ShR_SF/1
